simulink model "lab1sim"  (R2022a)
settings: Solver=ode45  StartTime=0.0  StopTime=2  FixedStep=0.001  RelTol=1e-3
values from neighbouring files (symbols this model uses):
  C = lC    [initlab1sim.m]
  dDZ = 0.1    [initlab1sim.m]
  DZPOS = 0    [initlab1sim.m]
  DZPOS_hat = 5    [initlab1sim.m]
  fixwidth = 2    [initlab1sim.m]
  GAM = lGAM    [initlab1sim.m]
  h = 0.001    [dfa.m]    (also in initlab1sim.m)
  K = lK    [initlab1sim.m]    (also in lqed.m = Phi*Kf+Kv)
  Lc = lLc    (= 1)    [initlab1sim.m]
  Le = lLe    [initlab1sim.m]
  OVERLAP = 0    [initlab1sim.m]
  PHI = lPHI    [initlab1sim.m]
  TL = + 1.3    (= 1.3)    [initlab1sim.m]
  TL_hat = + 1.3    (= 1.3)    [initlab1sim.m]
  TU = - 1.0    (= -1)    [initlab1sim.m]
  TU_hat = - 1.0    (= -1)    [initlab1sim.m]
  USE_FIX = 0    [fix_opencfg.m]    (also in initlab1sim.m)
undefined symbols (not defined in the file or in its folder): DiscIntNeverNeededParam, SimDen, SimNum
libraries: simulink_extras x1
settings Model: ExtModeTrigMode=oneshot  ExtModeArmWhenConnect=off  Creator=x98jg  LastModifiedBy=30416
settings SolverCC: AlgebraicLoopSolver=TrustRegion
settings DataIOCC: SaveFormat=Array  SignalLoggingSaveFormat=ModelDataLogs  ReturnWorkspaceOutputs=off
settings OptimizationCC: BooleanDataType=off  ExpressionDepthLimit=2147483647  LifeSpan=inf
settings DebuggingCC: SaveWithParameterizedLinksMsg=none  UnderspecifiedInitializationDetection=Classic  MergeDetectMultiDrivingBlocksExec=none  SignalResolutionControl=TryResolveAllWithWarning  MultiTaskDSMMsg=warning  MultiTaskCondExecSysMsg=none  FcnCallInpInsideContextMsg=warning  UnconnectedInputMsg=warning  UnconnectedOutputMsg=warning  UnconnectedLineMsg=warning  StateNameClashWarn=warning  SFUnexpectedBacktrackingDiag=warning  SFNoUnconditionalDefaultTransitionDiag=warning  SFExecutionAtInitializationDiag=none  SFMachineParentedDataDiag=warning  ArithmeticOperatorsInVariantConditions=warning
settings HardwareCC: ProdBitPerPointer=32  ProdBitPerSizeT=32  ProdBitPerPtrDiffT=32  ProdLargestAtomicFloat=None  ProdIntDivRoundTo=Undefined  ProdEndianess=Unspecified  ProdWordSize=32  ProdHWDeviceType=32-bit Generic  TargetUnknown=on
settings ModelReferenceCC: PropagateSignalLabelsOutOfModel=off
settings SFSimCC: SimUseLocalCustomCode=off  CustomCodeUndefinedFunction=UseInterfaceOnly
settings RTWCC: RTWUseLocalCustomCode=off
settings CodeAppCC: StateflowObjectComments=on
settings GRTTargetCC: TargetLangStandard=C89/C90 (ANSI)  CombineOutputUpdateFcns=off  GRTInterface=on
settings ConfigComp: CovMetricSettings=dw  CovSaveCumulativeToWorkspaceVar=on  CovSaveSingleToWorkspaceVar=on  CovExternalEMLEnable=off

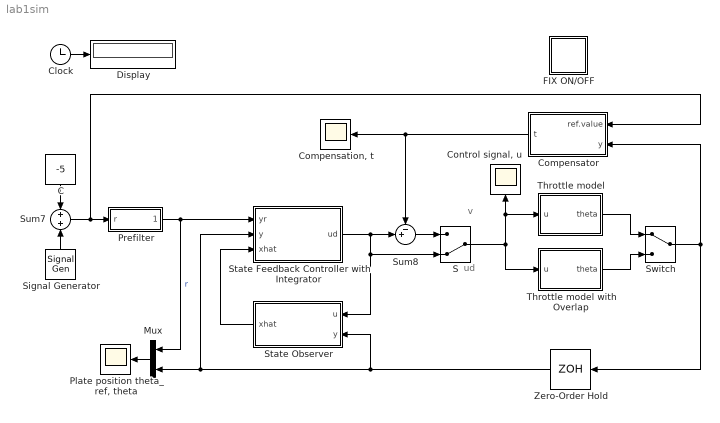
== system lab1sim ==
  note: v
  note: ud
  C : Constant  Value=-5
  Clock : Clock
  "Compensation, t" : Scope
  Compensator : Subsystem
  "Control signal, u" : Scope
  Display : Display
      settings: SampleTime=0.1
  FIX ON/OFF : Subsystem  Description=Fix ON/OFF
      settings: OpenFcn=fix_opencfg
      mask Display: disp('OFF')
  Mux : Mux  Inputs=2
  "Plate position theta_ref, theta" : Scope
  Prefilter : Subsystem
  S : ManualSwitch  CurrentSetting=0
  Signal Generator : SignalGenerator  WaveForm=square  Amplitude=5
  State Feedback Controller with Integrator : Subsystem
  State Observer : Subsystem
  Sum7 : Sum  InputSameDT=on  SaturateOnIntegerOverflow=on  OutDataTypeStr=Inherit: Same as first input
  Sum8 : Sum  Inputs=-+|  InputSameDT=on  SaturateOnIntegerOverflow=on  OutDataTypeStr=Inherit: Same as first input
  Switch : ManualSwitch
  Throttle model : Subsystem
  Throttle model with Overlap : Subsystem
  Zero-Order Hold : ZeroOrderHold  SampleTime=h
  wires:
  Signal Generator/1 -> Sum7/2
  Prefilter/1(rfiltered) -> Mux/1, State Feedback Controller with Integrator/1(yr)  "r"
  Mux/1 -> "Plate position theta_ref, theta"/1
  Zero-Order Hold/1 -> State Observer/2(y), Mux/2, State Feedback Controller with Integrator/2(y)
  State Observer/1(xhat) -> State Feedback Controller with Integrator/3(xhat)
  Sum7/1 -> Prefilter/1(r), Compensator/1(ref.value)
  Switch/1 -> Zero-Order Hold/1, Compensator/2(y)
  Sum8/1 -> S/1
  State Feedback Controller with Integrator/1(ud) -> Sum8/2, S/2, State Observer/1(u)
  Throttle model with Overlap/1(theta) -> Switch/2
  Throttle model/1(theta) -> Switch/1
  S/1 -> Throttle model/1(u), "Control signal, u"/1, Throttle model with Overlap/1(u)
  Compensator/1(t) -> Sum8/1, "Compensation, t"/1
  Clock/1 -> Display/1
  C/1 -> Sum7/1

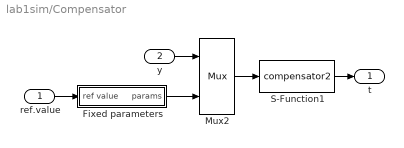
== system lab1sim/Compensator ==
  ref.value : Inport
  y : Inport  Port=2
  Fixed parameters : Subsystem
  Mux2 : Mux  Inputs=2
  S-Function1 : S-Function  FunctionName=compensator2  Parameters=h USE_FIX*fixwidth/2 -USE_FIX*fixwidth/2  SFunctionDeploymentMode=off  EnableBusSupport=off
  t : Outport
  wires:
  ref.value/1 -> Fixed parameters/1(ref value)
  y/1 -> Mux2/1
  Mux2/1 -> S-Function1/1
  S-Function1/1 -> t/1
  Fixed parameters/1(params) -> Mux2/2

== system lab1sim/FIX ON//OFF ==

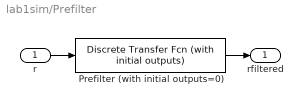
== system lab1sim/Prefilter ==
  r : Inport
  Prefilter (with initial outputs=0) : simulink_extras/Additional Discrete/Discrete Transfer Fcn (with initial outputs)  N=[21.3 1 -20.3]  D=[835 -1596 763]  U0=[0]  Y0=0  TS=h
      settings: SourceProductBaseCode=SL
  rfiltered : Outport
  wires:
  Prefilter (with initial outputs=0)/1 -> rfiltered/1
  r/1 -> Prefilter (with initial outputs=0)/1

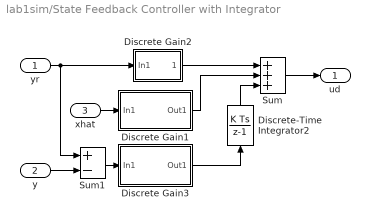
== system lab1sim/State Feedback Controller with Integrator ==
  yr : Inport
  y : Inport  Port=2
  xhat : Inport  Port=3
  Discrete Gain1 : Subsystem  mask(Discrete Gain){h=h, K=-Le(1:3)}
      mask prompts: h "Sample Time"; K "Gain"
      mask init:
      | s = get_param(gcb,'MaskValueString');
      | s = s(findstr(s,'|')+1:end);
      mask Display: disp(s)
  Discrete Gain2 : Subsystem  mask(Discrete Gain){h=h, K=Lc}
      mask prompts: h "Sample Time"; K "Gain"
      mask init:
      | s = get_param(gcb,'MaskValueString');
      | s = s(findstr(s,'|')+1:end);
      mask Display: disp(s)
  Discrete Gain3 : Subsystem  mask(Discrete Gain){h=h, K=-Le(4)}
      mask prompts: h "Sample Time"; K "Gain"
      mask init:
      | s = get_param(gcb,'MaskValueString');
      | s = s(findstr(s,'|')+1:end);
      mask Display: disp(s)
  Discrete-Time Integrator2 : DiscreteIntegrator  SampleTime=h  ICPrevOutput=DiscIntNeverNeededParam  ICPrevScaledInput=DiscIntNeverNeededParam
  Sum : Sum  Inputs=+++  InputSameDT=on  SaturateOnIntegerOverflow=on  OutDataTypeStr=Inherit: Same as first input
  Sum1 : Sum  Inputs=+-  InputSameDT=on  SaturateOnIntegerOverflow=on  OutDataTypeStr=Inherit: Same as first input
  ud : Outport
  wires:
  Discrete Gain1/1(Out1) -> Sum/2
  Discrete-Time Integrator2/1 -> Sum/3
  Sum/1 -> ud/1
  Discrete Gain3/1(Out1) -> Discrete-Time Integrator2/1
  Discrete Gain2/1(Out1) -> Sum/1
  xhat/1 -> Discrete Gain1/1(In1)
  y/1 -> Sum1/2
  yr/1 -> Discrete Gain2/1(In1), Sum1/1
  Sum1/1 -> Discrete Gain3/1(In1)

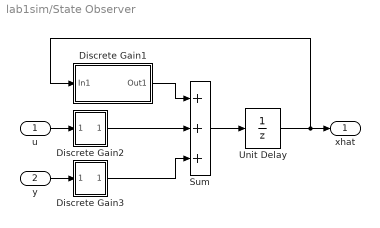
== system lab1sim/State Observer ==
  u : Inport
  y : Inport  Port=2
  Discrete Gain1 : Subsystem  mask(Discrete Gain){h=h, K=PHI-K*C}
      mask prompts: h "Sample Time"; K "Gain"
      mask init:
      | s = get_param(gcb,'MaskValueString');
      | s = s(findstr(s,'|')+1:end);
      mask Display: disp(s)
  Discrete Gain2 : Subsystem  mask(Discrete Gain){h=h, K=GAM}
      mask prompts: h "Sample Time"; K "Gain"
      mask init:
      | s = get_param(gcb,'MaskValueString');
      | s = s(findstr(s,'|')+1:end);
      mask Display: disp(s)
  Discrete Gain3 : Subsystem  mask(Discrete Gain){h=h, K=K}
      mask prompts: h "Sample Time"; K "Gain"
      mask init:
      | s = get_param(gcb,'MaskValueString');
      | s = s(findstr(s,'|')+1:end);
      mask Display: disp(s)
  Sum : Sum  Inputs=+++  InputSameDT=on  SaturateOnIntegerOverflow=on  OutDataTypeStr=Inherit: Same as first input
  Unit Delay : UnitDelay  SampleTime=h  HasFrameUpgradeWarning=on
  xhat : Outport
  wires:
  Discrete Gain1/1(Out1) -> Sum/1
  Discrete Gain2/1(Out1) -> Sum/2
  Discrete Gain3/1(Out1) -> Sum/3
  Sum/1 -> Unit Delay/1
  Unit Delay/1 -> Discrete Gain1/1(In1), xhat/1
  u/1 -> Discrete Gain2/1(In1)
  y/1 -> Discrete Gain3/1(In1)

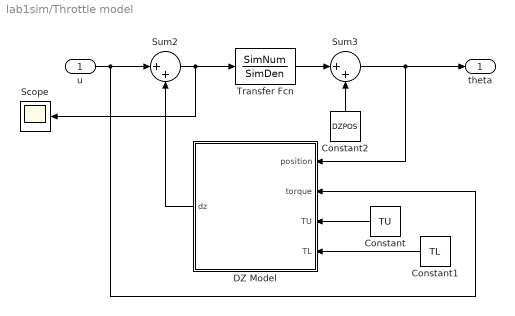
== system lab1sim/Throttle model ==
  u : Inport
  Constant : Constant  Value=TU
  Constant1 : Constant  Value=TL
  Constant2 : Constant  Value=DZPOS
  DZ Model : Subsystem
  Scope : Scope
  Sum2 : Sum  Inputs=|++  InputSameDT=on  SaturateOnIntegerOverflow=on  OutDataTypeStr=Inherit: Same as first input
  Sum3 : Sum  Inputs=|++  InputSameDT=on  SaturateOnIntegerOverflow=on  OutDataTypeStr=Inherit: Same as first input
  Transfer Fcn : TransferFcn  Numerator=SimNum  Denominator=SimDen
  theta : Outport
  wires:
  Sum3/1 -> DZ Model/1(position), theta/1
  Constant2/1 -> Sum3/2
  Transfer Fcn/1 -> Sum3/1
  u/1 -> DZ Model/2(torque), Sum2/1
  Constant/1 -> DZ Model/3(TU)
  Constant1/1 -> DZ Model/4(TL)
  Sum2/1 -> Transfer Fcn/1, Scope/1
  DZ Model/1(dz) -> Sum2/2

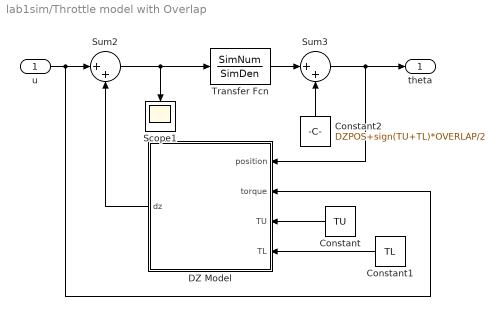
== system lab1sim/Throttle model with Overlap ==
  u : Inport
  Constant : Constant  Value=TU
  Constant1 : Constant  Value=TL
  Constant2 : Constant  Value=DZPOS+sign(TU+TL)*OVERLAP/2
  DZ Model : Subsystem
  Scope1 : Scope
  Sum2 : Sum  Inputs=|++  InputSameDT=on  SaturateOnIntegerOverflow=on  OutDataTypeStr=Inherit: Same as first input
  Sum3 : Sum  Inputs=|++  InputSameDT=on  SaturateOnIntegerOverflow=on  OutDataTypeStr=Inherit: Same as first input
  Transfer Fcn : TransferFcn  Numerator=SimNum  Denominator=SimDen
  theta : Outport
  wires:
  Sum3/1 -> DZ Model/1(position), theta/1
  Constant2/1 -> Sum3/2
  Transfer Fcn/1 -> Sum3/1
  Sum2/1 -> Scope1/1, Transfer Fcn/1
  Constant1/1 -> DZ Model/4(TL)
  Constant/1 -> DZ Model/3(TU)
  u/1 -> DZ Model/2(torque), Sum2/1
  DZ Model/1(dz) -> Sum2/2

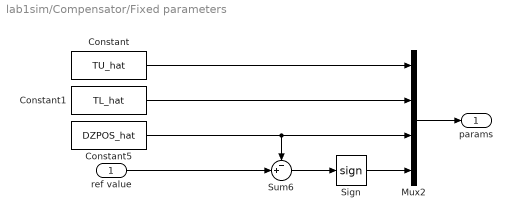
== system lab1sim/Compensator/Fixed parameters ==
  ref value : Inport
  Constant : Constant  Value=TU_hat
  Constant1 : Constant  Value=TL_hat
  Constant5 : Constant  Value=DZPOS_hat
  Mux2 : Mux
  Sign : Signum
  Sum6 : Sum  Inputs=-+|  InputSameDT=on  SaturateOnIntegerOverflow=on  OutDataTypeStr=Inherit: Same as first input
  params : Outport
  wires:
  Sign/1 -> Mux2/4
  Constant/1 -> Mux2/1
  ref value/1 -> Sum6/2
  Constant1/1 -> Mux2/2
  Mux2/1 -> params/1
  Sum6/1 -> Sign/1
  Constant5/1 -> Mux2/3, Sum6/1

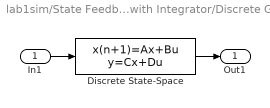
== system lab1sim/State Feedback Controller with Integrator/Discrete Gain1 ==
  In1 : Inport
  Discrete State-Space : DiscreteStateSpace  A=0  B=zeros(1,size(K,2))  C=zeros(size(K,1),1)  D=K  SampleTime=h
  Out1 : Outport
  wires:
  Discrete State-Space/1 -> Out1/1
  In1/1 -> Discrete State-Space/1

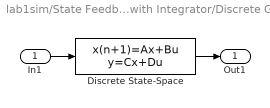
== system lab1sim/State Feedback Controller with Integrator/Discrete Gain2 ==
  In1 : Inport
  Discrete State-Space : DiscreteStateSpace  A=0  B=zeros(1,size(K,2))  C=zeros(size(K,1),1)  D=K  SampleTime=h
  Out1 : Outport
  wires:
  Discrete State-Space/1 -> Out1/1
  In1/1 -> Discrete State-Space/1

== system lab1sim/State Feedback Controller with Integrator/Discrete Gain3 ==
  In1 : Inport
  Discrete State-Space : DiscreteStateSpace  A=0  B=zeros(1,size(K,2))  C=zeros(size(K,1),1)  D=K  SampleTime=h
  Out1 : Outport
  wires:
  In1/1 -> Discrete State-Space/1
  Discrete State-Space/1 -> Out1/1

== system lab1sim/State Observer/Discrete Gain1 ==
  In1 : Inport
  Discrete State-Space : DiscreteStateSpace  A=0  B=zeros(1,size(K,2))  C=zeros(size(K,1),1)  D=K  SampleTime=h
  Out1 : Outport
  wires:
  Discrete State-Space/1 -> Out1/1
  In1/1 -> Discrete State-Space/1

== system lab1sim/State Observer/Discrete Gain2 ==
  In1 : Inport
  Discrete State-Space : DiscreteStateSpace  A=0  B=zeros(1,size(K,2))  C=zeros(size(K,1),1)  D=K  SampleTime=h
  Out1 : Outport
  wires:
  In1/1 -> Discrete State-Space/1
  Discrete State-Space/1 -> Out1/1

== system lab1sim/State Observer/Discrete Gain3 ==
  In1 : Inport
  Discrete State-Space : DiscreteStateSpace  A=0  B=zeros(1,size(K,2))  C=zeros(size(K,1),1)  D=K  SampleTime=h
  Out1 : Outport
  wires:
  Discrete State-Space/1 -> Out1/1
  In1/1 -> Discrete State-Space/1

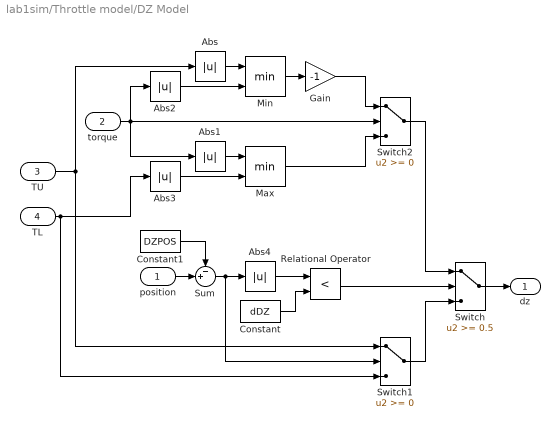
== system lab1sim/Throttle model/DZ Model ==
  position : Inport
  torque : Inport  Port=2
  TU : Inport  Port=3
  TL : Inport  Port=4
  Abs{,1..4} (5 alike) : Abs
  Constant : Constant  Value=dDZ
  Constant1 : Constant  Value=DZPOS
  Gain : Gain  Gain=-1  SaturateOnIntegerOverflow=on  OutDataTypeStr=Inherit: Same as input  ParamDataTypeStr=Inherit: Same as input
  Max : MinMax  Inputs=2  InputSameDT=on  SaturateOnIntegerOverflow=on
  Min : MinMax  Inputs=2  InputSameDT=on  SaturateOnIntegerOverflow=on
  Relational Operator : RelationalOperator  Operator=<
  Sum : Sum  Inputs=-+|  InputSameDT=on  SaturateOnIntegerOverflow=on  OutDataTypeStr=Inherit: Same as first input
  Switch : Switch  Threshold=0.5
  Switch1 : Switch
  Switch2 : Switch
  dz : Outport  InitialOutput=0
  wires:
  Abs4/1 -> Relational Operator/1
  Relational Operator/1 -> Switch/2
  Max/1 -> Switch2/3
  TL/1 -> Switch1/3, Abs3/1
  torque/1 -> Switch2/2, Abs1/1, Abs2/1
  TU/1 -> Switch1/1, Abs/1
  Abs/1 -> Min/1
  Abs1/1 -> Max/1
  Min/1 -> Gain/1
  Gain/1 -> Switch2/1
  Abs2/1 -> Min/2
  Abs3/1 -> Max/2
  Switch2/1 -> Switch/1
  Switch1/1 -> Switch/3
  Switch/1 -> dz/1
  Constant/1 -> Relational Operator/2
  position/1 -> Sum/2
  Constant1/1 -> Sum/1
  Sum/1 -> Abs4/1, Switch1/2

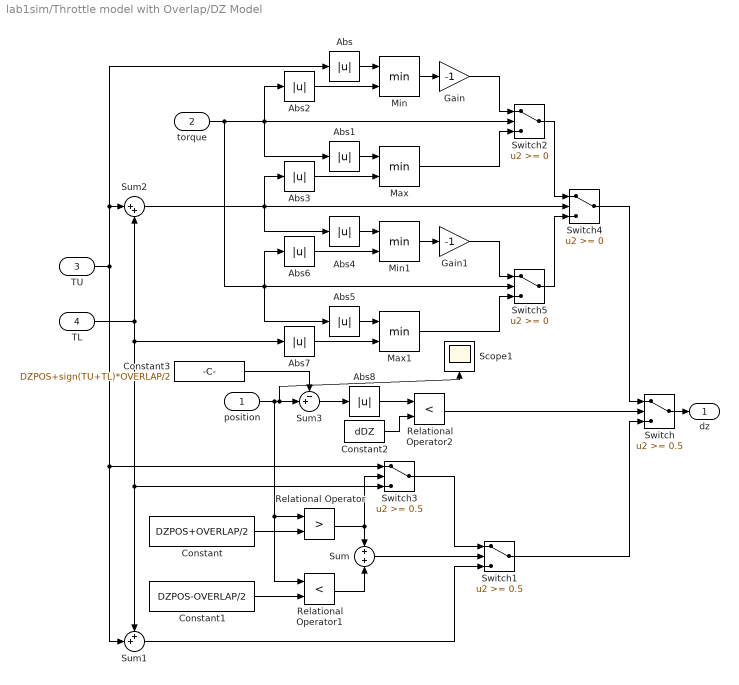
== system lab1sim/Throttle model with Overlap/DZ Model ==
  position : Inport
  torque : Inport  Port=2
  TU : Inport  Port=3
  TL : Inport  Port=4
  Abs{,1..8} (9 alike) : Abs
  Constant : Constant  Value=DZPOS+OVERLAP/2
  Constant1 : Constant  Value=DZPOS-OVERLAP/2
  Constant2 : Constant  Value=dDZ
  Constant3 : Constant  Value=DZPOS+sign(TU+TL)*OVERLAP/2
  Gain : Gain  Gain=-1  SaturateOnIntegerOverflow=on  OutDataTypeStr=Inherit: Same as input  ParamDataTypeStr=Inherit: Same as input
  Gain1 : Gain  Gain=-1  SaturateOnIntegerOverflow=on  OutDataTypeStr=Inherit: Same as input  ParamDataTypeStr=Inherit: Same as input
  Max : MinMax  Inputs=2  InputSameDT=on  SaturateOnIntegerOverflow=on
  Max1 : MinMax  Inputs=2  InputSameDT=on  SaturateOnIntegerOverflow=on
  Min : MinMax  Inputs=2  InputSameDT=on  SaturateOnIntegerOverflow=on
  Min1 : MinMax  Inputs=2  InputSameDT=on  SaturateOnIntegerOverflow=on
  Relational Operator : RelationalOperator  Operator=>
  Relational Operator1 : RelationalOperator  Operator=<
  Relational Operator2 : RelationalOperator  Operator=<
  Scope1 : Scope
  Sum : Sum  InputSameDT=on  SaturateOnIntegerOverflow=on  OutDataTypeStr=Inherit: Same as first input
  Sum1 : Sum  Inputs=++|  InputSameDT=on  SaturateOnIntegerOverflow=on  OutDataTypeStr=Inherit: Same as first input
  Sum2 : Sum  Inputs=|++  InputSameDT=on  SaturateOnIntegerOverflow=on  OutDataTypeStr=Inherit: Same as first input
  Sum3 : Sum  Inputs=-+|  InputSameDT=on  SaturateOnIntegerOverflow=on  OutDataTypeStr=Inherit: Same as first input
  Switch : Switch  Threshold=0.5
  Switch1 : Switch  Threshold=0.5
  Switch2 : Switch
  Switch3 : Switch  Threshold=0.5
  Switch4 : Switch
  Switch5 : Switch
  dz : Outport  InitialOutput=0
  wires:
  Abs8/1 -> Relational Operator2/1
  Relational Operator2/1 -> Switch/2
  Sum3/1 -> Abs8/1
  Constant2/1 -> Relational Operator2/2
  Constant3/1 -> Sum3/1
  position/1 -> Scope1/1, Sum3/2, Relational Operator/1, Relational Operator1/1
  TL/1 -> Sum2/2, Sum1/1, Switch3/3, Abs7/1
  TU/1 -> Switch3/1, Sum1/2, Sum2/1, Abs/1
  Abs/1 -> Min/1
  Abs1/1 -> Max/1
  Min/1 -> Gain/1
  Gain/1 -> Switch2/1
  Abs2/1 -> Min/2
  Abs3/1 -> Max/2
  Max1/1 -> Switch5/3
  Abs4/1 -> Min1/1
  Abs5/1 -> Max1/1
  Abs6/1 -> Min1/2
  Abs7/1 -> Max1/2
  Constant/1 -> Relational Operator/2
  Constant1/1 -> Relational Operator1/2
  Relational Operator1/1 -> Sum/2
  Sum/1 -> Switch1/2
  Sum1/1 -> Switch1/3
  Switch3/1 -> Switch1/1
  Relational Operator/1 -> Sum/1, Switch3/2
  Switch1/1 -> Switch/3
  torque/1 -> Switch2/2, Abs1/1, Abs2/1, Switch5/2, Abs6/1, Abs5/1
  Switch2/1 -> Switch4/1
  Switch5/1 -> Switch4/3
  Switch/1 -> dz/1
  Switch4/1 -> Switch/1
  Sum2/1 -> Switch4/2, Abs3/1, Abs4/1
  Max/1 -> Switch2/3
  Min1/1 -> Gain1/1
  Gain1/1 -> Switch5/1
